simulink model "ZN_cl_comparison_s"  (R2021b)
settings: Solver=VariableStepAuto  StartTime=0.0  StopTime=15  RelTol=1e-3
libraries: slpidlib x4
settings Model: Creator=nima8  LastModifiedBy=nima8

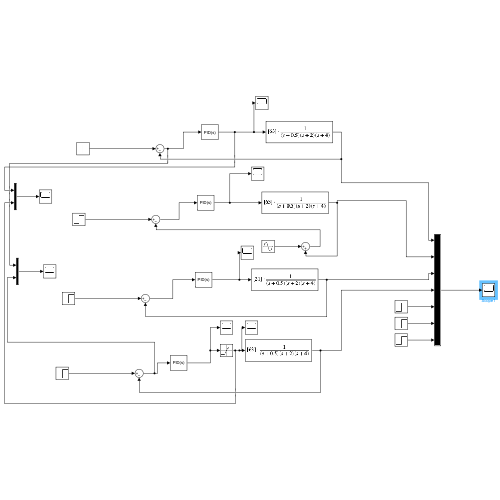
[thumbnail: Simulink's stored preview of the top-level diagram]
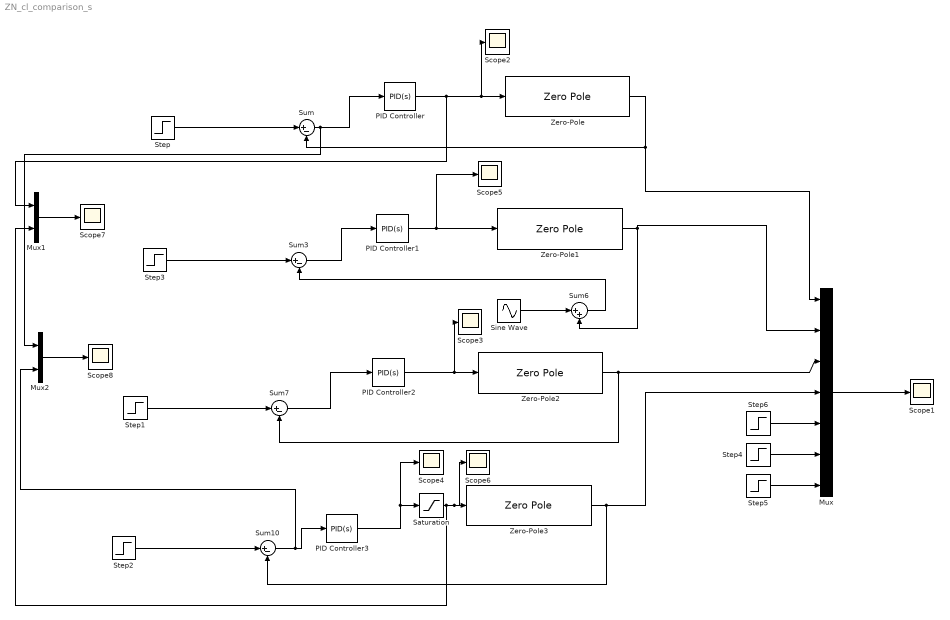
== system ZN_cl_comparison_s ==
  Mux : Mux  Inputs=7
  Mux1 : Mux  Inputs=2
  Mux2 : Mux  Inputs=2
  PID Controller{,1..3} (4 alike) : slpidlib/PID Controller  Controller=PID  Form=Ideal  TimeDomain=Continuous-time  UseExternalTs=off  SampleTime=-1  IntegratorMethod=Forward Euler  FilterMethod=Forward Euler  ControllerParametersSource=internal  P=0.6510  I=1.1450  D=0.2863  UseFilter=on  N=100  TunerSelectOption=Transfer Function Based (PID Tuner App)  InitialConditionSource=internal  InitialConditionForIntegrator=0  InitialConditionForFilter=0  DifferentiatorICPrevScaledInput=0  ExternalReset=none  TrackingMode=off  Kt=1  LimitOutput=off  SatLimitsSource=internal  UpperSaturationLimit=inf  LowerSaturationLimit=-inf  LinearizeAsGain=on  AntiWindupMode=none  Kb=1  POutMin=[]  POutMax=[]  IOutMin=[]  IOutMax=[]  DOutMin=[]  DOutMax=[]  NOutMin=[]  NOutMax=[]  SumOutMin=[]  SumOutMax=[]  SaturationOutMin=[]  SaturationOutMax=[]  PParamMin=[]  PParamMax=[]  IParamMin=[]  IParamMax=[]  DParamMin=[]  DParamMax=[]  NParamMin=[]  NParamMax=[]  KbParamMin=[]  KbParamMax=[]  KtParamMin=[]  KtParamMax=[]  KbOutMin=[]  KbOutMax=[]  KtOutMin=[]  KtOutMax=[]  IntegratorOutMin=[]  IntegratorOutMax=[]  FilterOutMin=[]  FilterOutMax=[]  SumI1OutMin=[]  SumI1OutMax=[]  SumI2OutMin=[]  SumI2OutMax=[]  SumI3OutMin=[]  SumI3OutMax=[]  SumI4OutMin=[]  SumI4OutMax=[]  SumDOutMin=[]  SumDOutMax=[]  DifferentiatorOutMin=[]  DifferentiatorOutMax=[]  FilterDiffOutCoefMin=[]  FilterDiffOutCoefMax=[]  ReciprocalOutMin=[]  ReciprocalOutMax=[]  SumDenOutMin=[]  SumDenOutMax=[]  SumNumOutMin=[]  SumNumOutMax=[]  DivideOutMin=[]  DivideOutMax=[]  UdiffTsProdOutMin=[]  UdiffTsProdOutMax=[]  NTsProdOutMin=[]  NTsProdOutMax=[]  UintegralTsProdOutMin=[]  UintegralTsProdOutMax=[]  UngainTsProdOutMin=[]  UngainTsProdOutMax=[]  IntegratorContinuousStateAttributes=''  IntegratorStateMustResolveToSignalObject=off  IntegratorRTWStateStorageClass=Auto  FilterContinuousStateAttributes=''  FilterStateMustResolveToSignalObject=off  FilterRTWStateStorageClass=Auto  ParallelPVariant=Passthrough  IdealPVariant=InternalParameters  IVariant=InternalParameters  DVariant=InternalParameters  IntegratorVariant=Continuous  SatVariant=Disabled  AWVariant=Passthrough  PCopyVariant=Disabled  TRVariant=Disabled  FdbkBlocksVariant=Forward  IdealPFdbkVariant=Disabled  SatFdbkVariant=Disabled  DerivativeFilterVariant=ContFilter  NVariant=InternalParameters  NCopyVariant=Disabled  FilterICVariant=InternalICsFilter  IntegratorICVariant=InternalICs  ExternalResetVariant=Disabled  TRSumVariant=Passthrough  SumFdbkVariant=Disabled  SumVariant=Sum_PID  TsampFilterVariant=InternalTs  TsampNgainVariant=Passthrough  TsampIntegralVariant=Passthrough  ExternalSaturationOutDataTypeStr=Inherit: Same as second input
  Saturation : Saturate  UpperLimit=14  LowerLimit=0.1
  Scope{1..8} (8 alike) : Scope
  Sine Wave : Sin  Amplitude=0.1  Frequency=60  SampleTime=0
  Step{,1..3,6} (5 alike) : Step  Time=0  SampleTime=0
  Step4 : Step  Time=0  After=0.98  SampleTime=0
  Step5 : Step  Time=0  After=1.02  SampleTime=0
  Sum{,3,7,10} (4 alike) : Sum  Inputs=|+-
  Sum6 : Sum  Inputs=|++
  Zero-Pole : ZeroPole  Zeros=[]  Poles=[-0.5 -2 -4]  Gain=[63]
  Zero-Pole1 : ZeroPole  Zeros=[]  Poles=[-0.5 -2 -4]  Gain=[63]
  Zero-Pole2 : ZeroPole  Zeros=[]  Poles=[-0.5 -2 -4]  Gain=[21]
  Zero-Pole3 : ZeroPole  Zeros=[]  Poles=[-0.5 -2 -4]  Gain=[63]
  wires:
  Step/1 -> Sum/1
  Zero-Pole/1 -> Sum/2, Mux/1
  PID Controller2/1 -> Zero-Pole2/1, Scope3/1
  Zero-Pole2/1 -> Sum7/2, Mux/3
  Step1/1 -> Sum7/1
  PID Controller3/1 -> Saturation/1, Scope4/1
  Zero-Pole1/1 -> Mux/2, Sum6/2
  Step3/1 -> Sum3/1
  Step6/1 -> Mux/5
  Zero-Pole3/1 -> Sum10/2, Mux/4
  Mux/1 -> Scope1/1
  Saturation/1 -> Scope6/1, Zero-Pole3/1, Mux1/2
  Sine Wave/1 -> Sum6/1
  Step4/1 -> Mux/6
  Step5/1 -> Mux/7
  Sum6/1 -> Sum3/2
  Step2/1 -> Sum10/1
  PID Controller/1 -> Mux1/1, Scope2/1, Zero-Pole/1
  Sum/1 -> Mux2/1, PID Controller/1
  PID Controller1/1 -> Zero-Pole1/1, Scope5/1
  Sum3/1 -> PID Controller1/1
  Sum7/1 -> PID Controller2/1
  Sum10/1 -> Mux2/2, PID Controller3/1
  Mux2/1 -> Scope8/1
  Mux1/1 -> Scope7/1
